simulink model "MAE272_HW5_Q4"  (R2023a)
settings: Solver=VariableStepAuto  StartTime=0.0  StopTime=10  RelTol=1e-3
settings Model: Creator=kaleb  LastModifiedBy=kaleb

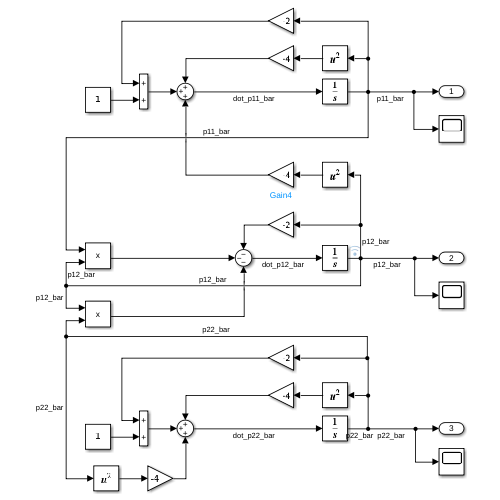
[thumbnail: Simulink's stored preview of the top-level diagram]
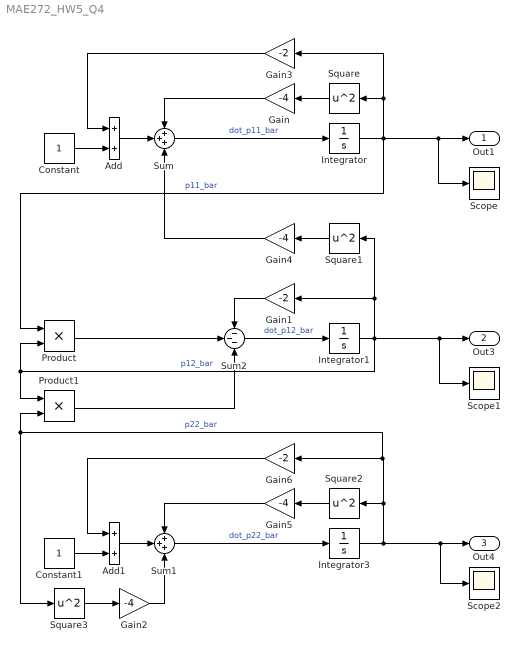
== system MAE272_HW5_Q4 ==
  Add : Sum
  Add1 : Sum
  Constant : Constant
  Constant1 : Constant
  Gain{,2,4..5} (4 alike) : Gain  Gain=-4
  Gain1 : Gain  Gain=-2
  Gain3 : Gain  Gain=-2
  Gain6 : Gain  Gain=-2
  Integrator : Integrator
  Integrator1 : Integrator
  Integrator3 : Integrator
  Product : Product
  Product1 : Product
  Scope : Scope
  Scope1 : Scope
  Scope2 : Scope
  Square{,1..3} (4 alike) : Math  Operator=square
  Sum : Sum  Inputs=+++
  Sum1 : Sum  Inputs=+++
  Sum2 : Sum  Inputs=---
  Out1 : Outport
  Out3 : Outport  Port=2
  Out4 : Outport  Port=3
  wires:
  Integrator/1 -> Gain3/1, Square/1, Scope/1, Out1/1, Product/1  "p11_bar"
  Gain/1 -> Sum/1
  Square/1 -> Gain/1
  Integrator1/1 -> Product/2, Product1/1, Scope1/1, Out3/1, Gain1/1, Square1/1  "p12_bar"
  Square1/1 -> Gain4/1
  Gain4/1 -> Sum/3
  Gain3/1 -> Add/1
  Constant/1 -> Add/2
  Add/1 -> Sum/2
  Sum/1 -> Integrator/1  "dot_p11_bar"
  Gain6/1 -> Add1/1
  Add1/1 -> Sum1/2
  Constant1/1 -> Add1/2
  Sum1/1 -> Integrator3/1  "dot_p22_bar"
  Gain5/1 -> Sum1/1
  Square2/1 -> Gain5/1
  Integrator3/1 -> Square3/1, Product1/2, Gain6/1, Square2/1, Scope2/1, Out4/1  "p22_bar"
  Product/1 -> Sum2/2
  Product1/1 -> Sum2/3
  Gain1/1 -> Sum2/1
  Sum2/1 -> Integrator1/1  "dot_p12_bar"
  Square3/1 -> Gain2/1
  Gain2/1 -> Sum1/3
